simulink model "xCoilPID"  (R2024a)
settings: Solver=VariableStepAuto  StartTime=0.0  StopTime=1000  RelTol=1e-3
undefined symbols (not defined in the file or in its folder): x
libraries: simulink x3
settings Model: Creator=b_ant  LastModifiedBy=b_ant
settings DataIOCC: SaveFormat=Array
settings DebuggingCC: UnconnectedInputMsg=warning  UnconnectedOutputMsg=warning  UnconnectedLineMsg=warning
settings ModelReferenceCC: EnableRefExpFcnMdlSchedulingChecks=on
settings RTWCC: GPUComputeCapability=3.5  DLArmComputeVersion=19.05

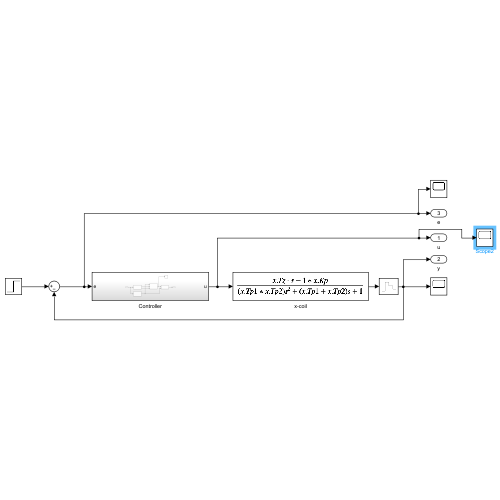
[thumbnail: Simulink's stored preview of the top-level diagram]
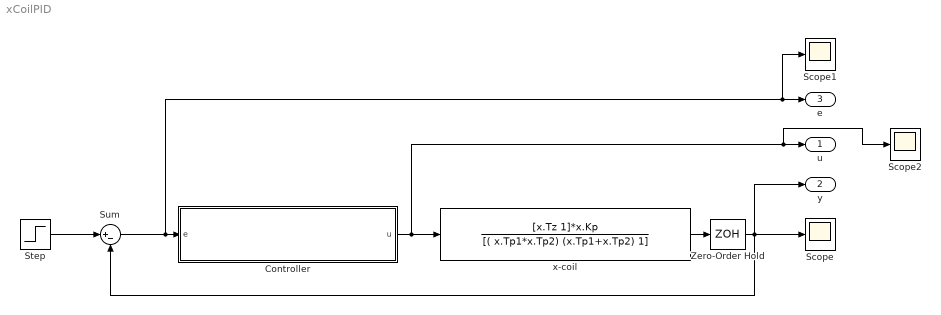
== system xCoilPID ==
  Controller : Subsystem
  Scope : Scope
  Scope1 : Scope
  Scope2 : Scope
  Step : Step  Time=0.001  SampleTime=0
  Sum : Sum  Inputs=|+-
  Zero-Order Hold : ZeroOrderHold
  x-coil : TransferFcn  Numerator=[x.Tz 1]*x.Kp  Denominator=[( x.Tp1*x.Tp2) (x.Tp1+x.Tp2) 1]
  u : Outport
  y : Outport  Port=2
  e : Outport  Port=3
  wires:
  Controller/1(u) -> Scope2/1, u/1, x-coil/1
  Sum/1 -> Scope1/1, e/1, Controller/1(e)
  x-coil/1 -> Zero-Order Hold/1
  Step/1 -> Sum/1
  Zero-Order Hold/1 -> Sum/2, y/1, Scope/1

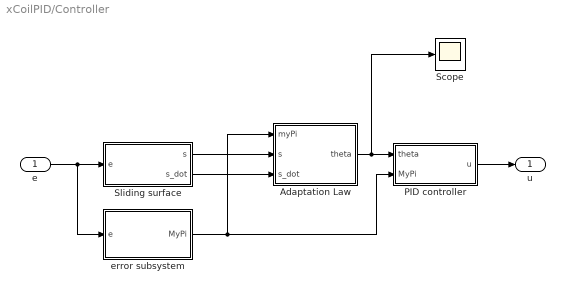
== system xCoilPID/Controller ==
  e : Inport
  Adaptation Law : Subsystem  mask{alpha=x.alpha, beta=x.beta, epsilon=x.epsilon, n=x.n, kd0=x.kd_init, ki0=x.ki_init, kp0=x.kp_init}
      mask prompts: kd0 "kd_0:"; ki0 "ki_0:"; kp0 "kp_0:"
      mask TypeOptions alpha: alpha/Value
      mask TypeOptions beta: beta/Value
      mask TypeOptions epsilon: epsilon/Value
      mask TypeOptions n: n/Value
      mask TypeOptions kd0: kd0/Value
      mask TypeOptions ki0: ki0/Value
      mask TypeOptions kp0: kp0/Value
  PID controller : Subsystem
  Scope : Scope
  Sliding surface : Subsystem  mask{Gain=x.lambda}
      mask prompts: Gain "Simulink:blkprm_prompts:GainGain"
      mask TypeOptions Gain: Gain/Gain
      mask DialogControl Gain Prompt: Gain:
  error subsystem : Subsystem
  u : Outport
  wires:
  Sliding surface/1(s) -> Adaptation Law/2(s)
  Sliding surface/2(s_dot) -> Adaptation Law/3(s_dot)
  PID controller/1(u) -> u/1
  Adaptation Law/1(theta) -> Scope/1, PID controller/1(theta)
  error subsystem/1(MyPi) -> PID controller/2(MyPi), Adaptation Law/1(myPi)
  e/1 -> error subsystem/1(e), Sliding surface/1(e)

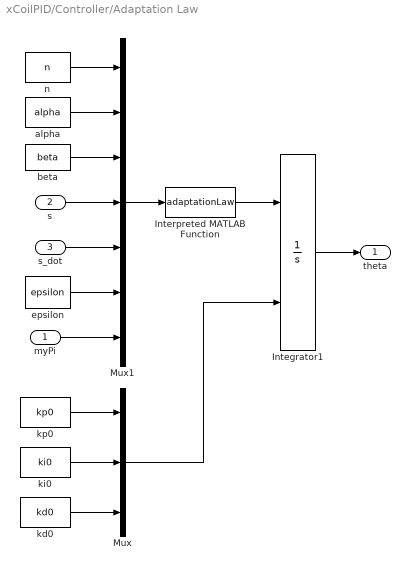
== system xCoilPID/Controller/Adaptation Law ==
  myPi : Inport
  s : Inport  Port=2
  s_dot : Inport  Port=3
  Integrator1 : Integrator  InitialConditionSource=external  InitialCondition=[1.460477259865257e-04,6.548069875818259e-05,0]
  Interpreted MATLAB Function : MATLABFcn  MATLABFcn=adaptationLaw
  Mux : Mux  Inputs=3
  Mux1 : Mux  Inputs=7
  alpha : Constant  Value=alpha
  beta : Constant  Value=beta
  epsilon : Constant  Value=epsilon
  kd0 : Constant  Value=kd0
  ki0 : Constant  Value=ki0
  kp0 : Constant  Value=kp0
  n : Constant  Value=n
  theta : Outport
  wires:
  alpha/1 -> Mux1/2
  Interpreted MATLAB Function/1 -> Integrator1/1
  myPi/1 -> Mux1/7
  s/1 -> Mux1/4
  epsilon/1 -> Mux1/6
  Integrator1/1 -> theta/1
  s_dot/1 -> Mux1/5
  beta/1 -> Mux1/3
  Mux1/1 -> Interpreted MATLAB Function/1
  n/1 -> Mux1/1
  ki0/1 -> Mux/2
  Mux/1 -> Integrator1/2
  kp0/1 -> Mux/1
  kd0/1 -> Mux/3

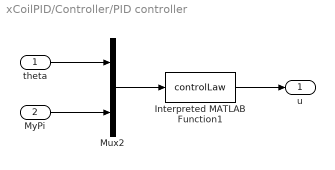
== system xCoilPID/Controller/PID controller ==
  theta : Inport
  MyPi : Inport  Port=2
  Interpreted MATLAB Function1 : MATLABFcn  MATLABFcn=controlLaw  OutputDimensions=1
  Mux2 : Mux  Inputs=2
  u : Outport
  wires:
  Mux2/1 -> Interpreted MATLAB Function1/1
  theta/1 -> Mux2/1
  Interpreted MATLAB Function1/1 -> u/1
  MyPi/1 -> Mux2/2

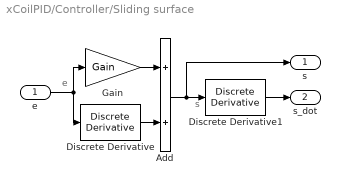
== system xCoilPID/Controller/Sliding surface ==
  note: s
  note: e
  e : Inport
  Add : Sum
  Discrete Derivative : simulink/Discrete/Discrete Derivative  gainval=1.0  ICPrevScaledInput=0.0  OutMin=[]  OutMax=[]  OutDataType=fixdt(1, 16)  OutScaling=2^-10  DoSatur=off
  Discrete Derivative1 : simulink/Discrete/Discrete Derivative  gainval=1.0  ICPrevScaledInput=0.0  OutMin=[]  OutMax=[]  OutDataType=fixdt(1, 16)  OutScaling=2^-10  DoSatur=off
  Gain : Gain  Gain=Gain
  s : Outport
  s_dot : Outport  Port=2
  wires:
  Add/1 -> Discrete Derivative1/1, s/1
  Gain/1 -> Add/1
  e/1 -> Gain/1, Discrete Derivative/1
  Discrete Derivative/1 -> Add/2
  Discrete Derivative1/1 -> s_dot/1

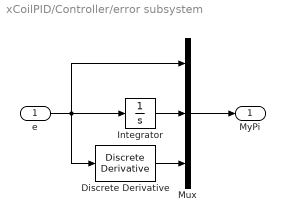
== system xCoilPID/Controller/error subsystem ==
  e : Inport
  Discrete Derivative : simulink/Discrete/Discrete Derivative  gainval=1.0  ICPrevScaledInput=0.0  OutMin=[]  OutMax=[]  OutDataType=fixdt(1, 16)  OutScaling=2^-10  DoSatur=off
  Integrator : Integrator
  Mux : Mux  Inputs=3
  MyPi : Outport
  wires:
  e/1 -> Mux/1, Discrete Derivative/1, Integrator/1
  Integrator/1 -> Mux/2
  Mux/1 -> MyPi/1
  Discrete Derivative/1 -> Mux/3
